simulink model "a2"  (R2015b)
settings: Solver=VariableStepAuto  StartTime=0.0  StopTime=500.0  RelTol=1e-3
settings Model: Creator=Admin  LastModifiedBy=Admin

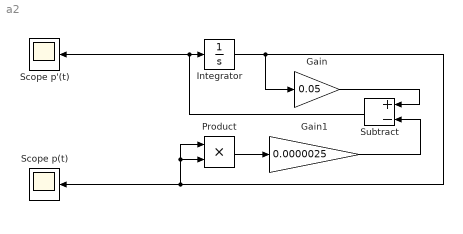
== system a2 ==
  Gain : Gain  Gain=0.05
  Gain1 : Gain  Gain=0.0000025
  Integrator : Integrator  InitialCondition=10000
  Product : Product
  Scope p'(t) : Scope
  Scope p(t) : Scope
  Subtract : Sum  Inputs=+-
  wires:
  Integrator/1 -> Product/1, Product/2, Scope p(t)/1, Gain/1
  Subtract/1 -> Scope p'(t)/1, Integrator/1
  Gain/1 -> Subtract/1
  Gain1/1 -> Subtract/2
  Product/1 -> Gain1/1
